simulink model "PS4_rst_example_ship_discrete"  (R2014b)
settings: Solver=ode45  StartTime=0.0  StopTime=10.0  RelTol=1e-3
values from neighbouring files (symbols this model uses):
  a = 0.8    [AW_5_2.m]    (also in PS4_ship_heading_RST_3h_script.m = 0.9; PS4_ship_heading_RST_noaa_script.m = 0.003; PS4_ship_heading_RST_script.m = 0.003; hw5.m = -2)
  h = findobj(gcf,'Type','line')    [AW_5_3.m]    (also in L4_RST_spring16.m = 0.1; PS4_ship_heading_RST_3h_script.m = 0.2; PS4_ship_heading_RST_noaa_script.m = 0.2; PS4_ship_heading_RST_script.m = 0.2)
  r1 = double(subs(sol.r1, vars, vals))    [AW_5_2.m]    (also in L4_RST_spring16.m = -0.856007930368168*a_d + 0.143992069631831; RST_example_spring18.m = params(1); hw5.m = -0.878368264722988*ea + 0.115597706410771)
  s0 = double(subs(sol.s0, vars, vals))    [AW_5_2.m]    (also in L4_RST_spring16.m = -28.7984139263664*a_d + 32.9380169529651; RST_example_spring18.m = params(2); hw5.m = -1.34327624390048*ea + 1.52396058689998)
  s1 = double(subs(sol.s1, vars, vals))    [AW_5_2.m]    (also in L4_RST_spring16.m = 24.6588108997672*a_d - 28.7984139263663; RST_example_spring18.m = params(3); hw5.m = 0.972399357505391*ea - 1.15308370050492)
  t0 = subs(Acs, z, 1) / subs(Bsa, z, 1)    [AW_5_3.m]    (also in L4_RST_spring16.m = 4.1396030266; RST_example_spring18.m = 0.210526315789; RST_sym.m = subs(Ac, z, 1) / subs(B, z, 1); RST_sym_handout.m = subs(Ac, z, 1) / subs(B, z, 1))
undefined symbols (not defined in the file or in its folder): r2, r3, s2, s3
libraries: simulink x1
settings Model: Creator=kjartan  LastModifiedBy=kjartan

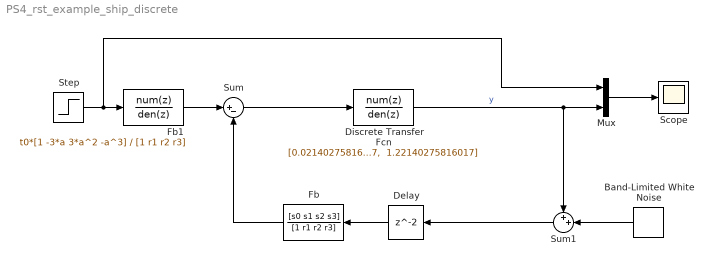
== system PS4_rst_example_ship_discrete ==
  Band-Limited White Noise : simulink/Sources/Band-Limited White Noise  Cov=[0.001]  Ts=0.1  seed=[23341]
  Delay : Delay  SampleTime=h
  Discrete Transfer Fcn : DiscreteTransferFcn  Numerator=[0.0214027581601699, 0.022877793471864]  Denominator="[1.0, - 2.22140275816017,  1.22140275816017]"  SampleTime=h
  Fb : DiscreteTransferFcn  Numerator=[s0 s1 s2 s3]  Denominator=[1 r1 r2 r3]  SampleTime=h
  Fb1 : DiscreteTransferFcn  Numerator=t0*[1 -3*a 3*a^2 -a^3]  Denominator=[1 r1 r2 r3]  SampleTime=h
  Mux : Mux  Inputs=2
  Scope : Scope
  Step : Step  SampleTime=0
  Sum : Sum  Inputs=|+-
  Sum1 : Sum  Inputs=++|
  wires:
  Sum/1 -> Discrete Transfer Fcn/1
  Sum1/1 -> Delay/1
  Fb/1 -> Sum/2
  Fb1/1 -> Sum/1
  Discrete Transfer Fcn/1 -> Sum1/1, Mux/2  "y"
  Mux/1 -> Scope/1
  Step/1 -> Mux/1, Fb1/1
  Band-Limited White Noise/1 -> Sum1/2
  Delay/1 -> Fb/1
